simulink model "FullyConnectedMMG"  (R2020b)
settings: Solver=ode3  StartTime=0.0  StopTime=TimeS  FixedStep=Ts  RelTol=1e-3
values from neighbouring files (symbols this model uses):
  fr = 60    [MMG_Parameters.m]
  Lgs = 600e-6    (= 0.0006)    [MMG_Parameters.m]
  MaxWind = 18    [MMG_Parameters.m]
  MicroVol = 575    [MMG_Parameters.m]
  MinWind = 3    [MMG_Parameters.m]
  NomVol = 600    [MMG_Parameters.m]
  NomWind = 10    [MMG_Parameters.m]
  Pnombb = 400    [MMG_Parameters.m]
  PnomDG = 150e3    (= 150000)    [MMG_Parameters.m]
  PnomWT = 400e3    (= 400000)    [MMG_Parameters.m]
  Rgs = 20e-6    (= 2e-05)    [MMG_Parameters.m]
  RtCapM1 = (5.1)*1e-1    (= 0.51)    [MMG_Parameters.m]
  RtCapM2 = (5.1)*1e-1    (= 0.51)    [MMG_Parameters.m]
  SOC = [70,80,75,65]    [MMG_Parameters.m]
  Ts = 8e-4    (= 0.0008)    [MMG_Parameters.m]    (also in SolveMONO.m = 0.005)
  Vgrid = 25e3    (= 25000)    [MMG_Parameters.m]
  VMic = 575    [MMG_Parameters.m]
  Vs = 120e3    (= 120000)    [MMG_Parameters.m]
undefined symbols (not defined in the file or in its folder): DiscIntNeverNeededParam
libraries: powerlib x64, simulink x24, powerlib_meascontrol x16
(part 3 of 5)

== system FullyConnectedMMG/Subsystem1/Microgrid 2/Variable Load1 ==
  Active Power Dynamics : Subsystem  VariantControl=T6NotZero
      mask Display: disp('1 / (1 + s T_P)','texmode','on');
  Dynamic Load Control : Subsystem
  Load2 : powerlib/Elements/Three-Phase Series RLC Load  LConnTagsString=A|B|C  Configuration=Y (grounded)  NominalVoltage=575  Vabc=[1e3 1e3 1e3]  Vabcp=[1e3 1e3 1e3]  NominalFrequency=60  UnbalancedPower=off  ActivePower=1e3  InductivePower=0  CapacitivePower=0  Pabc=[10e3 9e3 11e3]  QLabc=[100 90 110]  QCabc=[100 90 110]  Pabcp=[10e3 9e3 11e3]  QLabcp=[100 90 110]  QCabcp=[100 90 110]  Measurements=None  LoadType=constant Z
      settings: AttributesFormatString=P = %<ActivePower> W
  Simple Three-Phase Load : powerlib/Elements/Three-Phase Dynamic Load  NominalVoltage=[Vn Fn]  ActiveReactivePowers=[10000 15883.1]  PositiveSequence=[0.999844 -0.0038635]  ExternalControl=on  NpNq=[1.3 2]  TimeConstants="[0  0  0  0]"  MinimumVoltage=0.7  Tfilter=1e-2  LoadFlowParameters=[4,0,0,0,0]
      link override Model/Discrete 3-phase PLL: Ts=Ts
      link override Model/Discrete 3-phase PLL/Discrete PI Controller: Ts=Ts
      link override Model/Discrete 3-phase PLL/Discrete Rate Limiter: Ts=Ts
      link override Model/Discrete 3-phase PLL/Discrete Variable Frequency Mean value: Ts=Ts
      link override Model/Discrete 3-phase PLL/Discrete  2nd-Order Filter: Ts=Ts
      link override Model/Mean (Variable Frequency): Ts=Ts
      link override Model/Mean (Variable Frequency)1: Ts=Ts
      settings: SourceProductBaseCode=PS
  Sum1 : Sum  Inputs=|++
  Terminator : Terminator
  A : PMIOPort  Side=Right
  B : PMIOPort  Port=2  Side=Right
  C : PMIOPort  Port=3  Side=Right
  wires:
  Simple Three-Phase Load/1 -> Terminator/1
  Dynamic Load Control/1(PQ) -> Simple Three-Phase Load/1
  Sum1/1 -> Active Power Dynamics/1(In)
  Active Power Dynamics/1(Out) -> Dynamic Load Control/1(P0)
  [shPM2] -> Sum1/1
  [rePM2] -> Sum1/2
  connections:
  Simple Three-Phase Load/LConn1 -- Load2/LConn1 -- A/RConn1
  Simple Three-Phase Load/LConn3 -- C/RConn1 -- Load2/LConn3
  Simple Three-Phase Load/LConn2 -- Load2/LConn2 -- B/RConn1

== system FullyConnectedMMG/Subsystem1/Microgrid 1/Energy Storage/Charge Limits ==
  SOC (%) : Inport
  Pin : Inport  Port=2
  Qin : Inport  Port=3
  Overcharge Check : Subsystem
  Undercharge Check : Subsystem
  Pbatt : Outport  VectorParamsAs1DForOutWhenUnconnected=off
  Qbatt : Outport  Port=2  VectorParamsAs1DForOutWhenUnconnected=off
  wires:
  SOC (%)/1 -> Overcharge Check/1(SOC (%)), Undercharge Check/1(SOC (%))
  Undercharge Check/2(Qout) -> Qbatt/1
  Pin/1 -> Overcharge Check/2(Pin)
  Overcharge Check/1(Pout) -> Undercharge Check/2(Pin)
  Qin/1 -> Overcharge Check/3(Qin)
  Undercharge Check/1(Pout) -> Pbatt/1  "Pbatt"
  Overcharge Check/2(Qout) -> Undercharge Check/3(Qin)

== system FullyConnectedMMG/Subsystem1/Microgrid 1/Energy Storage/Reactive Power Capability ==
  Pin : Inport
  Qin : Inport  Port=2
  Constant : Constant  Value=Pnom
  Math Function : Math  Operator=square  SignedPower=on  SaturateOnIntegerOverflow=on
  Math Function1 : Math  Operator=square  SignedPower=on  SaturateOnIntegerOverflow=on
  Saturation Dynamic : simulink/Discontinuities/Saturation Dynamic  OutMin=[]  OutMax=[]  OutDataTypeStr=Inherit: Same as second input  OutDataType=fixdt(1, 16)  OutScaling=2^-10  DoSatur=off
  Sqrt : Sqrt  SaturateOnIntegerOverflow=on
  Sum : Sum  Inputs=-+|
  Unary Minus : UnaryMinus
  Qout : Outport  VectorParamsAs1DForOutWhenUnconnected=off
  wires:
  Sqrt/1 -> Saturation Dynamic/1, Unary Minus/1
  Math Function1/1 -> Sum/1
  Math Function/1 -> Sum/2
  Constant/1 -> Math Function/1
  Sum/1 -> Sqrt/1
  Unary Minus/1 -> Saturation Dynamic/3
  Saturation Dynamic/1 -> Qout/1
  Pin/1 -> Math Function1/1
  Qin/1 -> Saturation Dynamic/2

== system FullyConnectedMMG/Subsystem1/Microgrid 1/Energy Storage/Stored Energy Calculation (%) ==
  Pin : Inport
  Qin : Inport  Port=2
  Charge : Gain  Gain=Efficiency/100
  Compare To Zero : simulink/Logic and Bit Operations/Compare To Zero  relop=<=  OutDataTypeStr=boolean
  Constant : Constant  Value=kWh_Rated
  Discharge : Gain  Gain=1/(Efficiency/100)
  Divide : Product  Inputs=*/
  Gain3 : Gain  Gain=1/3600/1e3
  Gain5 : Gain  Gain=-1
  Integrator : Integrator  InitialCondition=(Initial_kWh_pc/100)*kWh_Rated*3600*1e3
  Math Function1 : Math  Operator=square  SignedPower=on  SaturateOnIntegerOverflow=on
  Math Function2 : Math  Operator=square  SignedPower=on  SaturateOnIntegerOverflow=on
  Product : Product
  Sign : Signum
  Sqrt : Sqrt  SaturateOnIntegerOverflow=on
  Sum : Sum  Inputs=|++
  Switch1 : Switch  Criteria=u2 ~= 0
  Transfer Fcn : TransferFcn  Denominator=[1 1]
  to % : Gain  Gain=100
  SE% : Outport  VectorParamsAs1DForOutWhenUnconnected=off
  wires:
  Sign/1 -> Product/1
  Sqrt/1 -> Product/2
  Sum/1 -> Sqrt/1
  Math Function2/1 -> Sum/2
  Math Function1/1 -> Sum/1
  Qin/1 -> Math Function2/1
  Pin/1 -> Math Function1/1, Sign/1
  Product/1 -> Transfer Fcn/1, Discharge/1, Charge/1
  Discharge/1 -> Switch1/3
  Gain5/1 -> Integrator/1
  to %/1 -> SE%/1
  Transfer Fcn/1 -> Compare To Zero/1
  Switch1/1 -> Gain5/1
  Gain3/1 -> Divide/1
  Constant/1 -> Divide/2
  Charge/1 -> Switch1/1
  Divide/1 -> to %/1
  Compare To Zero/1 -> Switch1/2
  Integrator/1 -> Gain3/1

== system FullyConnectedMMG/Subsystem1/Microgrid 1/Power Equation Wind Turbine (PQ Model)/Active Power Dynamics ==
  In : Inport
  1/Tp : Gain  Gain=1/0.004
  Discrete-Time Integrator : DiscreteIntegrator  Commented=on  SampleTime=-1  ICPrevOutput=DiscIntNeverNeededParam  ICPrevScaledInput=DiscIntNeverNeededParam
  Integrator : Integrator
  Sum : Sum  Inputs=|+-
  Out : Outport  VectorParamsAs1DForOutWhenUnconnected=off
  wires:
  Sum/1 -> 1/Tp/1
  In/1 -> Sum/1
  1/Tp/1 -> Integrator/1
  Integrator/1 -> Sum/2, Out/1

== system FullyConnectedMMG/Subsystem1/Microgrid 1/Power Equation Wind Turbine (PQ Model)/Reactive Power Dynamics ==
  In : Inport
  1/Tq : Gain  Gain=1/Tq
  Integrator : Integrator
  Sum : Sum  Inputs=|+-
  Out : Outport  VectorParamsAs1DForOutWhenUnconnected=off
  wires:
  Integrator/1 -> Out/1, Sum/2
  In/1 -> Sum/1
  1/Tq/1 -> Integrator/1
  Sum/1 -> 1/Tq/1

== system FullyConnectedMMG/Subsystem1/Microgrid 1/Power Equation Wind Turbine (PQ Model)/Wind Turbine Power Equation ==
  Wind (m/s) : Inport
  Constant : Constant  Value=Pselect
  Cubic Power with Cutoff : Subsystem
  Manufacturer Fit : Lookup_n-D  NumberOfTableDimensions=1  BreakpointsForDimension1=Uvec  Table=Pvec  ExtrapMethod=Clip  InternalRulePriority=Speed  RndMeth=Simplest  InputSameDT=on
  Multiport Switch : MultiPortSwitch
  Saturation : Saturate  UpperLimit=inf  LowerLimit=0  ZeroCross=off
      settings: AttributesFormatString=|
      | %<UpperLimit>
      | %<LowerLimit>
  Wind Turbine Properties : Subsystem
  Pwind : Outport  VectorParamsAs1DForOutWhenUnconnected=off
  wires:
  Wind (m/s)/1 -> Saturation/1
  Multiport Switch/1 -> Pwind/1
  Constant/1 -> Multiport Switch/1
  Saturation/1 -> Wind Turbine Properties/1(Wind (m/s)), Manufacturer Fit/1, Cubic Power with Cutoff/1(Wind (m/s))
  Cubic Power with Cutoff/1(Pwind) -> Multiport Switch/3
  Manufacturer Fit/1 -> Multiport Switch/4
  Wind Turbine Properties/1(Pwind) -> Multiport Switch/2

== system FullyConnectedMMG/Subsystem1/Microgrid 1/Simple Diesel Generator/Active Power Dynamics ==
  In : Inport
  1/Tp : Gain  Gain=1/0.004
  Discrete-Time Integrator : DiscreteIntegrator  Commented=on  SampleTime=-1  ICPrevOutput=DiscIntNeverNeededParam  ICPrevScaledInput=DiscIntNeverNeededParam
  Integrator : Integrator
  Sum : Sum  Inputs=|+-
  Out : Outport  VectorParamsAs1DForOutWhenUnconnected=off
  wires:
  Integrator/1 -> Out/1, Sum/2
  1/Tp/1 -> Integrator/1
  In/1 -> Sum/1
  Sum/1 -> 1/Tp/1

== system FullyConnectedMMG/Subsystem1/Microgrid 1/Simple Diesel Generator/Reactive Power Dynamics ==
  In : Inport
  1/Tq : Gain  Gain=1/Tq
  Integrator : Integrator
  Sum : Sum  Inputs=|+-
  Out : Outport  VectorParamsAs1DForOutWhenUnconnected=off
  wires:
  Sum/1 -> 1/Tq/1
  1/Tq/1 -> Integrator/1
  In/1 -> Sum/1
  Integrator/1 -> Sum/2, Out/1

== system FullyConnectedMMG/Subsystem1/Microgrid 1/Solar Array/Active Power Dynamics ==
  In : Inport
  1/Tp : Gain  Gain=1/0.004
  Discrete-Time Integrator : DiscreteIntegrator  Commented=on  SampleTime=-1  ICPrevOutput=DiscIntNeverNeededParam  ICPrevScaledInput=DiscIntNeverNeededParam
  Integrator : Integrator
  Sum : Sum  Inputs=|+-
  Out : Outport  VectorParamsAs1DForOutWhenUnconnected=off
  wires:
  Sum/1 -> 1/Tp/1
  In/1 -> Sum/1
  1/Tp/1 -> Integrator/1
  Integrator/1 -> Sum/2, Out/1

== system FullyConnectedMMG/Subsystem1/Microgrid 1/Variable Load/Active Power Dynamics ==
  In : Inport
  1/Tp : Gain  Gain=1/0.007
  Discrete-Time Integrator : DiscreteIntegrator  Commented=on  SampleTime=-1  ICPrevOutput=DiscIntNeverNeededParam  ICPrevScaledInput=DiscIntNeverNeededParam
  Integrator : Integrator
  Sum : Sum  Inputs=|+-
  Out : Outport  VectorParamsAs1DForOutWhenUnconnected=off
  wires:
  Sum/1 -> 1/Tp/1
  In/1 -> Sum/1
  Integrator/1 -> Sum/2, Out/1
  1/Tp/1 -> Integrator/1

== system FullyConnectedMMG/Subsystem1/Microgrid 1/Variable Load/Dynamic Load Control ==
  P0 : Inport
  Fcn : Fcn  Expr=sqrt(1/u(1)-1)
  Mux : Mux  Inputs=2
  Product : Product
  Summer1 : Constant  Value=PF
  PQ : Outport  VectorParamsAs1DForOutWhenUnconnected=off
  wires:
  Summer1/1 -> Fcn/1
  Fcn/1 -> Product/2
  P0/1 -> Product/1, Mux/1
  Mux/1 -> PQ/1
  Product/1 -> Mux/2  "Qo"

== system FullyConnectedMMG/Subsystem1/Microgrid 1/Variable Load1/Active Power Dynamics ==
  In : Inport
  1/Tp : Gain  Gain=1/0.007
  Discrete-Time Integrator : DiscreteIntegrator  Commented=on  SampleTime=-1  ICPrevOutput=DiscIntNeverNeededParam  ICPrevScaledInput=DiscIntNeverNeededParam
  Integrator : Integrator
  Sum : Sum  Inputs=|+-
  Out : Outport  VectorParamsAs1DForOutWhenUnconnected=off
  wires:
  Sum/1 -> 1/Tp/1
  In/1 -> Sum/1
  Integrator/1 -> Sum/2, Out/1
  1/Tp/1 -> Integrator/1

== system FullyConnectedMMG/Subsystem1/Microgrid 1/Variable Load1/Dynamic Load Control ==
  P0 : Inport
  Fcn : Fcn  Expr=sqrt(1/u(1)-1)
  Mux : Mux  Inputs=2
  Product : Product
  Summer1 : Constant  Value=PF
  PQ : Outport  VectorParamsAs1DForOutWhenUnconnected=off
  wires:
  Summer1/1 -> Fcn/1
  Fcn/1 -> Product/2
  P0/1 -> Product/1, Mux/1
  Mux/1 -> PQ/1
  Product/1 -> Mux/2  "Qo"

== system FullyConnectedMMG/Subsystem1/Microgrid 2/Energy Storage/Charge Limits ==
  SOC (%) : Inport
  Pin : Inport  Port=2
  Qin : Inport  Port=3
  Overcharge Check : Subsystem
  Undercharge Check : Subsystem
  Pbatt : Outport  VectorParamsAs1DForOutWhenUnconnected=off
  Qbatt : Outport  Port=2  VectorParamsAs1DForOutWhenUnconnected=off
  wires:
  SOC (%)/1 -> Overcharge Check/1(SOC (%)), Undercharge Check/1(SOC (%))
  Undercharge Check/2(Qout) -> Qbatt/1
  Pin/1 -> Overcharge Check/2(Pin)
  Overcharge Check/1(Pout) -> Undercharge Check/2(Pin)
  Qin/1 -> Overcharge Check/3(Qin)
  Undercharge Check/1(Pout) -> Pbatt/1  "Pbatt"
  Overcharge Check/2(Qout) -> Undercharge Check/3(Qin)

== system FullyConnectedMMG/Subsystem1/Microgrid 2/Energy Storage/Reactive Power Capability ==
  Pin : Inport
  Qin : Inport  Port=2
  Constant : Constant  Value=Pnom
  Math Function : Math  Operator=square  SignedPower=on  SaturateOnIntegerOverflow=on
  Math Function1 : Math  Operator=square  SignedPower=on  SaturateOnIntegerOverflow=on
  Saturation Dynamic : simulink/Discontinuities/Saturation Dynamic  OutMin=[]  OutMax=[]  OutDataTypeStr=Inherit: Same as second input  OutDataType=fixdt(1, 16)  OutScaling=2^-10  DoSatur=off
  Sqrt : Sqrt  SaturateOnIntegerOverflow=on
  Sum : Sum  Inputs=-+|
  Unary Minus : UnaryMinus
  Qout : Outport  VectorParamsAs1DForOutWhenUnconnected=off
  wires:
  Sqrt/1 -> Saturation Dynamic/1, Unary Minus/1
  Math Function1/1 -> Sum/1
  Math Function/1 -> Sum/2
  Constant/1 -> Math Function/1
  Sum/1 -> Sqrt/1
  Unary Minus/1 -> Saturation Dynamic/3
  Saturation Dynamic/1 -> Qout/1
  Pin/1 -> Math Function1/1
  Qin/1 -> Saturation Dynamic/2

== system FullyConnectedMMG/Subsystem1/Microgrid 2/Energy Storage/Stored Energy Calculation (%) ==
  Pin : Inport
  Qin : Inport  Port=2
  Charge : Gain  Gain=Efficiency/100
  Compare To Zero : simulink/Logic and Bit Operations/Compare To Zero  relop=<=  OutDataTypeStr=boolean
  Constant : Constant  Value=kWh_Rated
  Discharge : Gain  Gain=1/(Efficiency/100)
  Divide : Product  Inputs=*/
  Gain3 : Gain  Gain=1/3600/1e3
  Gain5 : Gain  Gain=-1
  Integrator : Integrator  InitialCondition=(Initial_kWh_pc/100)*kWh_Rated*3600*1e3
  Math Function1 : Math  Operator=square  SignedPower=on  SaturateOnIntegerOverflow=on
  Math Function2 : Math  Operator=square  SignedPower=on  SaturateOnIntegerOverflow=on
  Product : Product
  Sign : Signum
  Sqrt : Sqrt  SaturateOnIntegerOverflow=on
  Sum : Sum  Inputs=|++
  Switch1 : Switch  Criteria=u2 ~= 0
  Transfer Fcn : TransferFcn  Denominator=[1 1]
  to % : Gain  Gain=100
  SE% : Outport  VectorParamsAs1DForOutWhenUnconnected=off
  wires:
  Sign/1 -> Product/1
  Sqrt/1 -> Product/2
  Sum/1 -> Sqrt/1
  Math Function2/1 -> Sum/2
  Math Function1/1 -> Sum/1
  Qin/1 -> Math Function2/1
  Pin/1 -> Math Function1/1, Sign/1
  Product/1 -> Transfer Fcn/1, Discharge/1, Charge/1
  Discharge/1 -> Switch1/3
  Gain5/1 -> Integrator/1
  to %/1 -> SE%/1
  Transfer Fcn/1 -> Compare To Zero/1
  Switch1/1 -> Gain5/1
  Gain3/1 -> Divide/1
  Constant/1 -> Divide/2
  Charge/1 -> Switch1/1
  Divide/1 -> to %/1
  Compare To Zero/1 -> Switch1/2
  Integrator/1 -> Gain3/1

== system FullyConnectedMMG/Subsystem1/Microgrid 2/Power Equation Wind Turbine (PQ Model)1/Active Power Dynamics ==
  In : Inport
  1/Tp : Gain  Gain=1/0.004
  Integrator : Integrator
  Sum : Sum  Inputs=|+-
  Out : Outport  VectorParamsAs1DForOutWhenUnconnected=off
  wires:
  Sum/1 -> 1/Tp/1
  1/Tp/1 -> Integrator/1
  In/1 -> Sum/1
  Integrator/1 -> Sum/2, Out/1

== system FullyConnectedMMG/Subsystem1/Microgrid 2/Power Equation Wind Turbine (PQ Model)1/Reactive Power Dynamics ==
  In : Inport
  1/Tq : Gain  Gain=1/Tq
  Integrator : Integrator
  Sum : Sum  Inputs=|+-
  Out : Outport  VectorParamsAs1DForOutWhenUnconnected=off
  wires:
  Integrator/1 -> Out/1, Sum/2
  In/1 -> Sum/1
  1/Tq/1 -> Integrator/1
  Sum/1 -> 1/Tq/1

== system FullyConnectedMMG/Subsystem1/Microgrid 2/Power Equation Wind Turbine (PQ Model)1/Wind Turbine Power Equation ==
  Wind (m/s) : Inport
  Constant : Constant  Value=Pselect
  Cubic Power with Cutoff : Subsystem
  Manufacturer Fit : Lookup_n-D  NumberOfTableDimensions=1  BreakpointsForDimension1=Uvec  Table=Pvec  ExtrapMethod=Clip  InternalRulePriority=Speed  RndMeth=Simplest  InputSameDT=on
  Multiport Switch : MultiPortSwitch
  Saturation : Saturate  UpperLimit=inf  LowerLimit=0  ZeroCross=off
      settings: AttributesFormatString=|
      | %<UpperLimit>
      | %<LowerLimit>
  Wind Turbine Properties : Subsystem
  Pwind : Outport  VectorParamsAs1DForOutWhenUnconnected=off
  wires:
  Wind (m/s)/1 -> Saturation/1
  Multiport Switch/1 -> Pwind/1
  Constant/1 -> Multiport Switch/1
  Saturation/1 -> Wind Turbine Properties/1(Wind (m/s)), Manufacturer Fit/1, Cubic Power with Cutoff/1(Wind (m/s))
  Cubic Power with Cutoff/1(Pwind) -> Multiport Switch/3
  Manufacturer Fit/1 -> Multiport Switch/4
  Wind Turbine Properties/1(Pwind) -> Multiport Switch/2

== system FullyConnectedMMG/Subsystem1/Microgrid 2/Simple Diesel Generator/Active Power Dynamics ==
  In : Inport
  1/Tp : Gain  Gain=1/0.004
  Discrete-Time Integrator : DiscreteIntegrator  Commented=on  SampleTime=-1  ICPrevOutput=DiscIntNeverNeededParam  ICPrevScaledInput=DiscIntNeverNeededParam
  Integrator : Integrator
  Sum : Sum  Inputs=|+-
  Out : Outport  VectorParamsAs1DForOutWhenUnconnected=off
  wires:
  Integrator/1 -> Out/1, Sum/2
  1/Tp/1 -> Integrator/1
  In/1 -> Sum/1
  Sum/1 -> 1/Tp/1

== system FullyConnectedMMG/Subsystem1/Microgrid 2/Simple Diesel Generator/Reactive Power Dynamics ==
  In : Inport
  1/Tq : Gain  Gain=1/Tq
  Integrator : Integrator
  Sum : Sum  Inputs=|+-
  Out : Outport  VectorParamsAs1DForOutWhenUnconnected=off
  wires:
  Sum/1 -> 1/Tq/1
  1/Tq/1 -> Integrator/1
  In/1 -> Sum/1
  Integrator/1 -> Sum/2, Out/1

== system FullyConnectedMMG/Subsystem1/Microgrid 2/Solar Array/Active Power Dynamics ==
  In : Inport
  1/Tp : Gain  Gain=1/0.004
  Discrete-Time Integrator : DiscreteIntegrator  Commented=on  SampleTime=-1  ICPrevOutput=DiscIntNeverNeededParam  ICPrevScaledInput=DiscIntNeverNeededParam
  Integrator : Integrator
  Sum : Sum  Inputs=|+-
  Out : Outport  VectorParamsAs1DForOutWhenUnconnected=off
  wires:
  Sum/1 -> 1/Tp/1
  In/1 -> Sum/1
  1/Tp/1 -> Integrator/1
  Integrator/1 -> Sum/2, Out/1

== system FullyConnectedMMG/Subsystem1/Microgrid 2/Variable Load/Active Power Dynamics ==
  In : Inport
  1/Tp : Gain  Gain=1/0.004
  Discrete-Time Integrator : DiscreteIntegrator  Commented=on  SampleTime=-1  ICPrevOutput=DiscIntNeverNeededParam  ICPrevScaledInput=DiscIntNeverNeededParam
  Integrator : Integrator
  Sum : Sum  Inputs=|+-
  Out : Outport  VectorParamsAs1DForOutWhenUnconnected=off
  wires:
  Sum/1 -> 1/Tp/1
  In/1 -> Sum/1
  1/Tp/1 -> Integrator/1
  Integrator/1 -> Sum/2, Out/1

== system FullyConnectedMMG/Subsystem1/Microgrid 2/Variable Load/Dynamic Load Control ==
  P0 : Inport
  Fcn : Fcn  Expr=sqrt(1/u(1)-1)
  Mux : Mux  Inputs=2
  Product : Product
  Summer1 : Constant  Value=PF
  PQ : Outport  VectorParamsAs1DForOutWhenUnconnected=off
  wires:
  Product/1 -> Mux/2  "Qo"
  Mux/1 -> PQ/1
  P0/1 -> Mux/1, Product/1
  Fcn/1 -> Product/2
  Summer1/1 -> Fcn/1

== system FullyConnectedMMG/Subsystem1/Microgrid 2/Variable Load1/Active Power Dynamics ==
  In : Inport
  1/Tp : Gain  Gain=1/0.007
  Discrete-Time Integrator : DiscreteIntegrator  Commented=on  SampleTime=-1  ICPrevOutput=DiscIntNeverNeededParam  ICPrevScaledInput=DiscIntNeverNeededParam
  Integrator : Integrator
  Sum : Sum  Inputs=|+-
  Out : Outport  VectorParamsAs1DForOutWhenUnconnected=off
  wires:
  Sum/1 -> 1/Tp/1
  In/1 -> Sum/1
  Integrator/1 -> Sum/2, Out/1
  1/Tp/1 -> Integrator/1

== system FullyConnectedMMG/Subsystem1/Microgrid 2/Variable Load1/Dynamic Load Control ==
  P0 : Inport
  Fcn : Fcn  Expr=sqrt(1/u(1)-1)
  Mux : Mux  Inputs=2
  Product : Product
  Summer1 : Constant  Value=PF
  PQ : Outport  VectorParamsAs1DForOutWhenUnconnected=off
  wires:
  Summer1/1 -> Fcn/1
  Fcn/1 -> Product/2
  P0/1 -> Product/1, Mux/1
  Mux/1 -> PQ/1
  Product/1 -> Mux/2  "Qo"

== system FullyConnectedMMG/Subsystem1/Microgrid 1/Energy Storage/Charge Limits/Overcharge Check ==
  SOC (%) : Inport
  Pin : Inport  Port=2
  Qin : Inport  Port=3
  Backlash : Backlash  BacklashWidth=1e-3  InitialOutput=Initial_kWh_pc  ZeroCross=off
  Compare To Constant : simulink/Logic and Bit Operations/Compare To Constant  relop=>  const=UpChrgLim  OutDataTypeStr=boolean
  Compare To Zero : simulink/Logic and Bit Operations/Compare To Zero  relop=<=  OutDataTypeStr=boolean
  Constant : Constant  Value=0
  Constant1 : Constant  Value=0
  Logical Operator : Logic  AllPortsSameDT=off  OutDataTypeStr=boolean
  Switch : Switch  Criteria=u2 ~= 0
  Switch1 : Switch  Criteria=u2 ~= 0
  Pout : Outport  VectorParamsAs1DForOutWhenUnconnected=off
  Qout : Outport  Port=2  VectorParamsAs1DForOutWhenUnconnected=off
  wires:
  Backlash/1 -> Compare To Constant/1
  Switch1/1 -> Qout/1
  Constant1/1 -> Switch1/1
  Qin/1 -> Switch1/3
  Compare To Zero/1 -> Logical Operator/2
  Switch/1 -> Pout/1
  Pin/1 -> Switch/3, Compare To Zero/1
  SOC (%)/1 -> Backlash/1
  Constant/1 -> Switch/1
  Logical Operator/1 -> Switch/2, Switch1/2
  Compare To Constant/1 -> Logical Operator/1

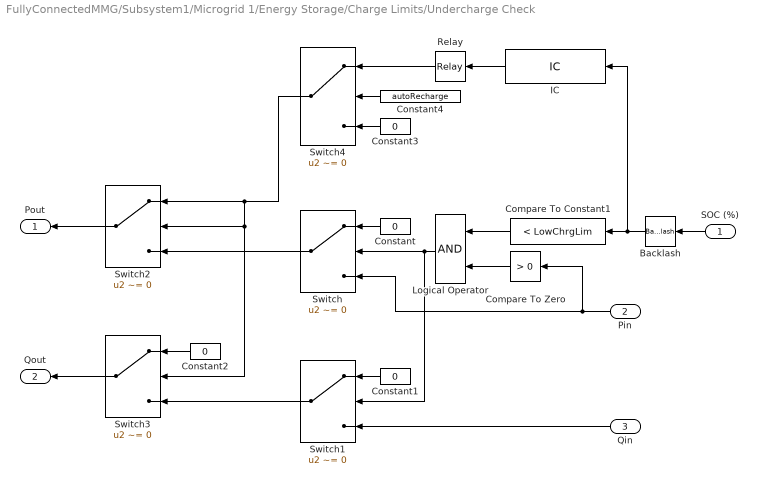
== system FullyConnectedMMG/Subsystem1/Microgrid 1/Energy Storage/Charge Limits/Undercharge Check ==
  SOC (%) : Inport
  Pin : Inport  Port=2
  Qin : Inport  Port=3
  Backlash : Backlash  BacklashWidth=1e-3  InitialOutput=Initial_kWh_pc  ZeroCross=off
  Compare To Constant1 : simulink/Logic and Bit Operations/Compare To Constant  relop=<  const=LowChrgLim  OutDataTypeStr=boolean
  Compare To Zero : simulink/Logic and Bit Operations/Compare To Zero  relop=>  OutDataTypeStr=boolean
  Constant{,1..3} (4 alike) : Constant  Value=0
  Constant4 : Constant  Value=autoRecharge
  IC : InitialCondition  Value=RechargeSOC
  Logical Operator : Logic  AllPortsSameDT=off  OutDataTypeStr=boolean
  Relay : Relay  OnSwitchValue=RechargeSOC  OffSwitchValue=LowChrgLim  OnOutputValue=0  OffOutputValue=-Precharge/100*Pnom
  Switch{,1..4} (5 alike) : Switch  Criteria=u2 ~= 0
  Pout : Outport  VectorParamsAs1DForOutWhenUnconnected=off
  Qout : Outport  Port=2  VectorParamsAs1DForOutWhenUnconnected=off
  wires:
  Constant4/1 -> Switch4/2
  Constant3/1 -> Switch4/3
  Relay/1 -> Switch4/1
  Constant2/1 -> Switch3/1
  Switch1/1 -> Switch3/3
  Switch3/1 -> Qout/1
  Switch2/1 -> Pout/1
  Switch/1 -> Switch2/3
  IC/1 -> Relay/1
  Switch4/1 -> Switch3/2, Switch2/2, Switch2/1
  Backlash/1 -> Compare To Constant1/1, IC/1
  Qin/1 -> Switch1/3
  Constant1/1 -> Switch1/1
  Compare To Constant1/1 -> Logical Operator/1
  Logical Operator/1 -> Switch1/2, Switch/2
  Constant/1 -> Switch/1
  SOC (%)/1 -> Backlash/1
  Pin/1 -> Compare To Zero/1, Switch/3
  Compare To Zero/1 -> Logical Operator/2

== system FullyConnectedMMG/Subsystem1/Microgrid 1/Power Equation Wind Turbine (PQ Model)/Wind Turbine Power Equation/Cubic Power with Cutoff ==
  Wind (m/s) : Inport
  A : Gain  Gain=Pnom/(Unom^3 - Umin^3)
  B : Bias  Bias=-Pnom/(Unom^3 - Umin^3)*Umin^3
  Compare To Constant : simulink/Logic and Bit Operations/Compare To Constant  relop=<  const=Umin  OutDataTypeStr=boolean
  Compare To Constant1 : simulink/Logic and Bit Operations/Compare To Constant  relop=>  const=Umax  OutDataTypeStr=boolean
  Compare To Constant2 : simulink/Logic and Bit Operations/Compare To Constant  relop=<  const=Unom  OutDataTypeStr=boolean
  Logical Operator : Logic  Operator=OR  AllPortsSameDT=off  OutDataTypeStr=boolean
  Math Function : Math  Operator=pow  SignedPower=on  SaturateOnIntegerOverflow=on
  Max Power : Constant  Value=Pnom
  No Power : Constant  Value=0
  No Power1 : Constant  Value=3
  Switch : Switch  Criteria=u2 ~= 0  ZeroCross=off
  Switch1 : Switch  Criteria=u2 ~= 0  ZeroCross=off
  Pwind : Outport  VectorParamsAs1DForOutWhenUnconnected=off
  wires:
  B/1 -> Switch1/1
  Compare To Constant2/1 -> Switch1/2
  Compare To Constant1/1 -> Logical Operator/2
  Math Function/1 -> A/1
  No Power1/1 -> Math Function/2
  No Power/1 -> Switch/1
  Switch1/1 -> Switch/3
  Max Power/1 -> Switch1/3
  Wind (m/s)/1 -> Compare To Constant/1, Compare To Constant1/1, Math Function/1, Compare To Constant2/1
  A/1 -> B/1
  Logical Operator/1 -> Switch/2
  Switch/1 -> Pwind/1
  Compare To Constant/1 -> Logical Operator/1

== system FullyConnectedMMG/Subsystem1/Microgrid 1/Power Equation Wind Turbine (PQ Model)/Wind Turbine Power Equation/Wind Turbine Properties ==
  Wind (m/s) : Inport
  Compare To Constant : simulink/Logic and Bit Operations/Compare To Constant  relop=<  const=Umin  OutDataTypeStr=boolean
  Compare To Constant1 : simulink/Logic and Bit Operations/Compare To Constant  relop=>  const=Umax  OutDataTypeStr=boolean
  Compare To Constant2 : simulink/Logic and Bit Operations/Compare To Constant  relop=<  const=Unom  OutDataTypeStr=boolean
  Logical Operator : Logic  Operator=OR  AllPortsSameDT=off  OutDataTypeStr=boolean
  Max Power : Constant  Value=Pnom
  No Power : Constant  Value=0
  Properties : Subsystem
  Switch : Switch  Criteria=u2 ~= 0  ZeroCross=off
  Switch1 : Switch  Criteria=u2 ~= 0  ZeroCross=off
  Pwind : Outport  VectorParamsAs1DForOutWhenUnconnected=off
  wires:
  Compare To Constant/1 -> Logical Operator/1
  Switch/1 -> Pwind/1
  Logical Operator/1 -> Switch/2
  Wind (m/s)/1 -> Compare To Constant2/1, Properties/1(In1), Compare To Constant1/1, Compare To Constant/1
  Max Power/1 -> Switch1/3
  Switch1/1 -> Switch/3
  No Power/1 -> Switch/1
  Compare To Constant1/1 -> Logical Operator/2
  Compare To Constant2/1 -> Switch1/2
  Properties/1(Out1) -> Switch1/1

== system FullyConnectedMMG/Subsystem1/Microgrid 2/Energy Storage/Charge Limits/Overcharge Check ==
  SOC (%) : Inport
  Pin : Inport  Port=2
  Qin : Inport  Port=3
  Backlash : Backlash  BacklashWidth=1e-3  InitialOutput=Initial_kWh_pc  ZeroCross=off
  Compare To Constant : simulink/Logic and Bit Operations/Compare To Constant  relop=>  const=UpChrgLim  OutDataTypeStr=boolean
  Compare To Zero : simulink/Logic and Bit Operations/Compare To Zero  relop=<=  OutDataTypeStr=boolean
  Constant : Constant  Value=0
  Constant1 : Constant  Value=0
  Logical Operator : Logic  AllPortsSameDT=off  OutDataTypeStr=boolean
  Switch : Switch  Criteria=u2 ~= 0
  Switch1 : Switch  Criteria=u2 ~= 0
  Pout : Outport  VectorParamsAs1DForOutWhenUnconnected=off
  Qout : Outport  Port=2  VectorParamsAs1DForOutWhenUnconnected=off
  wires:
  Backlash/1 -> Compare To Constant/1
  Switch1/1 -> Qout/1
  Constant1/1 -> Switch1/1
  Qin/1 -> Switch1/3
  Compare To Zero/1 -> Logical Operator/2
  Switch/1 -> Pout/1
  Pin/1 -> Switch/3, Compare To Zero/1
  SOC (%)/1 -> Backlash/1
  Constant/1 -> Switch/1
  Logical Operator/1 -> Switch/2, Switch1/2
  Compare To Constant/1 -> Logical Operator/1

== system FullyConnectedMMG/Subsystem1/Microgrid 2/Energy Storage/Charge Limits/Undercharge Check ==
  SOC (%) : Inport
  Pin : Inport  Port=2
  Qin : Inport  Port=3
  Backlash : Backlash  BacklashWidth=1e-3  InitialOutput=Initial_kWh_pc  ZeroCross=off
  Compare To Constant1 : simulink/Logic and Bit Operations/Compare To Constant  relop=<  const=LowChrgLim  OutDataTypeStr=boolean
  Compare To Zero : simulink/Logic and Bit Operations/Compare To Zero  relop=>  OutDataTypeStr=boolean
  Constant{,1..3} (4 alike) : Constant  Value=0
  Constant4 : Constant  Value=autoRecharge
  IC : InitialCondition  Value=RechargeSOC
  Logical Operator : Logic  AllPortsSameDT=off  OutDataTypeStr=boolean
  Relay : Relay  OnSwitchValue=RechargeSOC  OffSwitchValue=LowChrgLim  OnOutputValue=0  OffOutputValue=-Precharge/100*Pnom
  Switch{,1..4} (5 alike) : Switch  Criteria=u2 ~= 0
  Pout : Outport  VectorParamsAs1DForOutWhenUnconnected=off
  Qout : Outport  Port=2  VectorParamsAs1DForOutWhenUnconnected=off
  wires:
  Constant4/1 -> Switch4/2
  Constant3/1 -> Switch4/3
  Relay/1 -> Switch4/1
  Constant2/1 -> Switch3/1
  Switch1/1 -> Switch3/3
  Switch3/1 -> Qout/1
  Switch2/1 -> Pout/1
  Switch/1 -> Switch2/3
  IC/1 -> Relay/1
  Switch4/1 -> Switch3/2, Switch2/2, Switch2/1
  Backlash/1 -> Compare To Constant1/1, IC/1
  Qin/1 -> Switch1/3
  Constant1/1 -> Switch1/1
  Compare To Constant1/1 -> Logical Operator/1
  Logical Operator/1 -> Switch1/2, Switch/2
  Constant/1 -> Switch/1
  SOC (%)/1 -> Backlash/1
  Pin/1 -> Compare To Zero/1, Switch/3
  Compare To Zero/1 -> Logical Operator/2

== system FullyConnectedMMG/Subsystem1/Microgrid 2/Power Equation Wind Turbine (PQ Model)1/Wind Turbine Power Equation/Cubic Power with Cutoff ==
  Wind (m/s) : Inport
  A : Gain  Gain=Pnom/(Unom^3 - Umin^3)
  B : Bias  Bias=-Pnom/(Unom^3 - Umin^3)*Umin^3
  Compare To Constant : simulink/Logic and Bit Operations/Compare To Constant  relop=<  const=Umin  OutDataTypeStr=boolean
  Compare To Constant1 : simulink/Logic and Bit Operations/Compare To Constant  relop=>  const=Umax  OutDataTypeStr=boolean
  Compare To Constant2 : simulink/Logic and Bit Operations/Compare To Constant  relop=<  const=Unom  OutDataTypeStr=boolean
  Logical Operator : Logic  Operator=OR  AllPortsSameDT=off  OutDataTypeStr=boolean
  Math Function : Math  Operator=pow  SignedPower=on  SaturateOnIntegerOverflow=on
  Max Power : Constant  Value=Pnom
  No Power : Constant  Value=0
  No Power1 : Constant  Value=3
  Switch : Switch  Criteria=u2 ~= 0  ZeroCross=off
  Switch1 : Switch  Criteria=u2 ~= 0  ZeroCross=off
  Pwind : Outport  VectorParamsAs1DForOutWhenUnconnected=off
  wires:
  B/1 -> Switch1/1
  Compare To Constant2/1 -> Switch1/2
  Compare To Constant1/1 -> Logical Operator/2
  Math Function/1 -> A/1
  No Power1/1 -> Math Function/2
  No Power/1 -> Switch/1
  Switch1/1 -> Switch/3
  Max Power/1 -> Switch1/3
  Wind (m/s)/1 -> Compare To Constant/1, Compare To Constant1/1, Math Function/1, Compare To Constant2/1
  A/1 -> B/1
  Logical Operator/1 -> Switch/2
  Switch/1 -> Pwind/1
  Compare To Constant/1 -> Logical Operator/1

== system FullyConnectedMMG/Subsystem1/Microgrid 2/Power Equation Wind Turbine (PQ Model)1/Wind Turbine Power Equation/Wind Turbine Properties ==
  Wind (m/s) : Inport
  Compare To Constant : simulink/Logic and Bit Operations/Compare To Constant  relop=<  const=Umin  OutDataTypeStr=boolean
  Compare To Constant1 : simulink/Logic and Bit Operations/Compare To Constant  relop=>  const=Umax  OutDataTypeStr=boolean
  Compare To Constant2 : simulink/Logic and Bit Operations/Compare To Constant  relop=<  const=Unom  OutDataTypeStr=boolean
  Logical Operator : Logic  Operator=OR  AllPortsSameDT=off  OutDataTypeStr=boolean
  Max Power : Constant  Value=Pnom
  No Power : Constant  Value=0
  Properties : Subsystem
  Switch : Switch  Criteria=u2 ~= 0  ZeroCross=off
  Switch1 : Switch  Criteria=u2 ~= 0  ZeroCross=off
  Pwind : Outport  VectorParamsAs1DForOutWhenUnconnected=off
  wires:
  Compare To Constant/1 -> Logical Operator/1
  Switch/1 -> Pwind/1
  Logical Operator/1 -> Switch/2
  Wind (m/s)/1 -> Compare To Constant2/1, Properties/1(In1), Compare To Constant1/1, Compare To Constant/1
  Max Power/1 -> Switch1/3
  Switch1/1 -> Switch/3
  No Power/1 -> Switch/1
  Compare To Constant1/1 -> Logical Operator/2
  Compare To Constant2/1 -> Switch1/2
  Properties/1(Out1) -> Switch1/1

== system FullyConnectedMMG/Subsystem1/Microgrid 1/Power Equation Wind Turbine (PQ Model)/Wind Turbine Power Equation/Wind Turbine Properties/Properties ==
  In1 : Inport
  Air Density : Gain  Gain=rho
  Blade Swept Area (m^2) : Gain  Gain=A
  Gain : Gain  Gain=1/2
  Power Coefficient : Constant  Value=Cp
  "Product " : Product  SaturateOnIntegerOverflow=on  OutDataTypeStr=Inherit: Same as first input
  wind_speed^3 : Fcn  Expr=u(1)^3
  Out1 : Outport  VectorParamsAs1DForOutWhenUnconnected=off
  wires:
  Gain/1 -> Blade Swept Area (m^2)/1
  "Product "/1 -> Out1/1
  Air Density/1 -> Gain/1
  In1/1 -> wind_speed^3/1
  Power Coefficient/1 -> "Product "/2
  wind_speed^3/1 -> Air Density/1
  Blade Swept Area (m^2)/1 -> "Product "/1

== system FullyConnectedMMG/Subsystem1/Microgrid 2/Power Equation Wind Turbine (PQ Model)1/Wind Turbine Power Equation/Wind Turbine Properties/Properties ==
  In1 : Inport
  Air Density : Gain  Gain=rho
  Blade Swept Area (m^2) : Gain  Gain=A
  Gain : Gain  Gain=1/2
  Power Coefficient : Constant  Value=Cp
  "Product " : Product  SaturateOnIntegerOverflow=on  OutDataTypeStr=Inherit: Same as first input
  wind_speed^3 : Fcn  Expr=u(1)^3
  Out1 : Outport  VectorParamsAs1DForOutWhenUnconnected=off
  wires:
  Gain/1 -> Blade Swept Area (m^2)/1
  "Product "/1 -> Out1/1
  Air Density/1 -> Gain/1
  In1/1 -> wind_speed^3/1
  Power Coefficient/1 -> "Product "/2
  wind_speed^3/1 -> Air Density/1
  Blade Swept Area (m^2)/1 -> "Product "/1
